simulink model "SCwith2SAs2aug"  (R2025b)
settings: Solver=VariableStepAuto  StartTime=0.0  StopTime=10.0  RelTol=1e-3
undefined symbols (not defined in the file or in its folder): DAP0, InvDyn, Jr, sig4, uls, ureal, uss, uw, XI
libraries: RCTblocks x77
(part 1 of 2)
settings Model: Creator=d.alazard  LastModifiedBy=andre
settings SolverCC: AlgebraicLoopSolver=TrustRegion
settings DebuggingCC: AlgebraicLoopMsg=none  UnconnectedInputMsg=warning  UnconnectedOutputMsg=warning  UnconnectedLineMsg=warning
settings ModelReferenceCC: EnableRefExpFcnMdlSchedulingChecks=on
settings RTWCC: GPUComputeCapability=3.5  DLArmComputeVersion=19.05

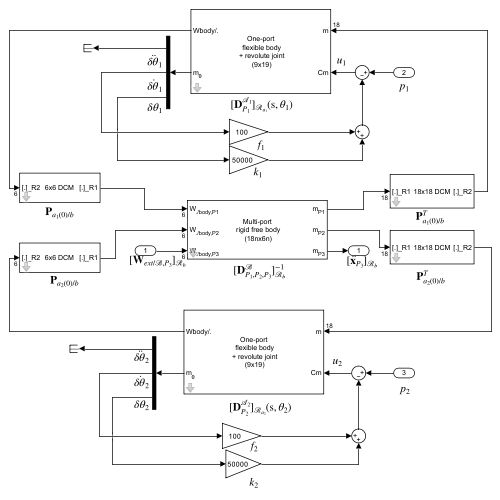
[thumbnail: Simulink's stored preview of the top-level diagram]
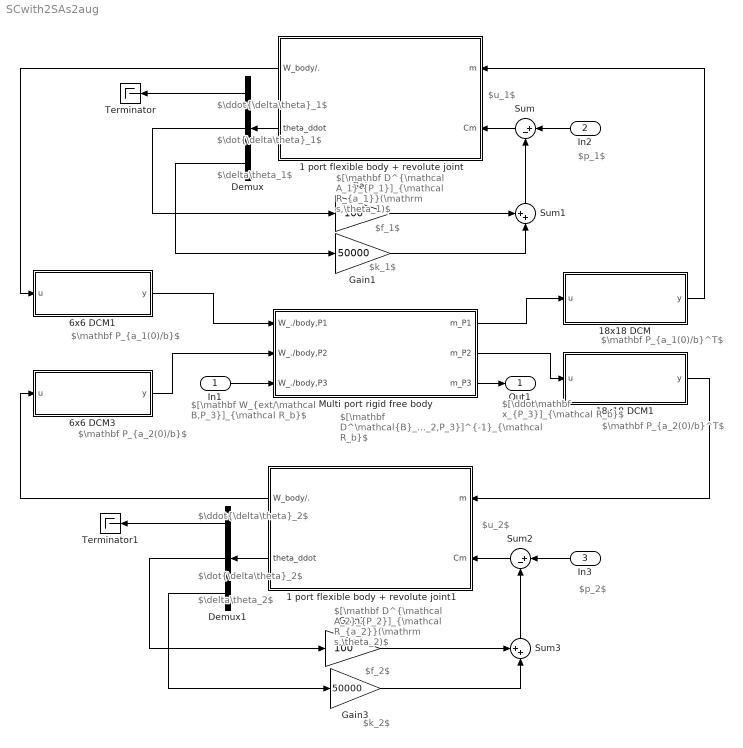
== system SCwith2SAs2aug ==
  note: $[\ddot\mathbf x_{P_3}]_{\mathcal R_b}$
  note: $u_1$
  note: $\ddot{\delta\theta}_1$
  note: $\mathbf P_{a_1(0)/b}^T$
  note: $[\mathbf D^\mathcal{B}_{P_1,P_2,P_3}]^{-1}_{\mathcal R_b}$
  note: $\mathbf P_{a_1(0)/b}$
  note: $\mathbf P_{a_2(0)/b}$
  note: $\mathbf P_{a_2(0)/b}^T$
  note: $\dot{\delta\theta}_1$
  note: $\dot{\delta\theta}_2$
  note: $\ddot{\delta\theta}_2$
  note: $\delta\theta_1$
  note: $\delta\theta_2$
  note: $p_1$
  note: $u_2$
  note: $p_2$
  note: $f_1$
  note: $k_1$
  note: $k_2$
  note: $f_2$
  note: $[\mathbf D^{\mathcal A_1}_{P_1}]_{\mathcal R_{a_1}}(\mathrm s,\theta_1)$
  note: $[\mathbf D^{\mathcal A_2}_{P_2}]_{\mathcal R_{a_2}}(\mathrm s,\theta_2)$
  note: $[\mathbf W_{ext/\mathcal B,P_3}]_{\mathcal R_b}$
  In1 : Inport
  In2 : Inport  Port=2
  In3 : Inport  Port=3
  1 port flexible body + revolute joint : Subsystem  mask(One-port flexibe body with revolute joint (9x19)){m=43, Ig=[17 0 0;0 62 0;0 0 79], OG=[2.07;0;0], OP=[0;0;0], ra=[1;0;0], theta=ureal('Theta',0,'Range',[-pi pi]), n=3, xi=0.005, w1=ureal('w1',5.6,'percent',20), L11=0, L12=0, L13=-5.12, L14=0, L15=12.5, L16=0, w2=ureal('w2',19.3,'percent',20), L21=0, L22=0, L23=0, L24=-3.84, L25=0, L26=0, w3=ureal('w3',35.4,'percent',20), L31=0, L32=0, L33=-2.97, L34=0, L35=2.51, L36=0, w4=2.83*2*pi, L41=0.0004, L42=-0.9132, L43=2.7900, L44=-1.8763, L45=-0.0246, L46=0.0031, w5=4.30*2*pi, L51=-0.0053, L52=5.878, L53=-1.0144, L54=3.0180, L55=-0.0124, L56=-0.0001, w6=0, L61=0, L62=0, L63=0, L64=0, L65=0, L66=0, w7=0, L71=0, L72=0, L73=0, L74=0, L75=0, L76=0, w8=0, L81=0, L82=0, L83=0, L84=0, L85=0, L86=0, w9=0, L91=0, L92=0, L93=0, L94=0, L95=0, L96=0, w10=0, L101=0, L102=0, L103=0, L104=0, L105=0, L106=0}
      mask prompts: m "Mass (Kg)"; Ig "Inertia (at G in Ra, Kgm^2)"; OG "OG (3x1 vector in Ra, m)"; OP "OP (3x1 vector in Ra, m)"; ra "ra (joint axis) (3x1 vector)"; theta "Angular configuration (rad)"; n "Number of flexible modes"; xi "Common damping ratio"; w1 "Frequency (rd/s)"; L11 "Tx (Kg^0.5)"; L12 "Ty (Kg^0.5)"; L13 "Tz (Kg^0.5)"; L14 "Rx (m.Kg^0.5)"; L15 "Ry (m.Kg^0.5)"; L16 "Rz (m.Kg^0.5)"; w2 "Frequency (rd/s)"; L21 "Tx (Kg^0.5)"; L22 "Ty (Kg^0.5)"; L23 "Tz (Kg^0.5)"; L24 "Rx (m.Kg^0.5)"; L25 "Ry (m.Kg^0.5)"; L26 "Rz (m.Kg^0.5)"; w3 "Frequency (rd/s)"; L31 "Tx (Kg^0.5)"; L32 "Ty (Kg^0.5)"; L33 "Tz (Kg^0.5)"; L34 "Rx (m.Kg^0.5)"; L35 "Ry (m.Kg^0.5)"; L36 "Rz (m.Kg^0.5)"; w4 "Frequency (rd/s)"; L41 "Tx (Kg^0.5)"; L42 "Ty (Kg^0.5)"; L43 "Tz (Kg^0.5)"; L44 "Rx (m.Kg^0.5)"; L45 "Ry (m.Kg^0.5)"; L46 "Rz (m.Kg^0.5)"; w5 "Frequency (rd/s)"; L51 "Tx (Kg^0.5)"; L52 "Ty (Kg^0.5)"; L53 "Tz (Kg^0.5)"; L54 "Rx (m.Kg^0.5)"; L55 "Ry (m.Kg^0.5)"; L56 "Rz (m.Kg^0.5)"; w6 "Frequency (rd/s)"; L61 "Tx (Kg^0.5)"; L62 "Ty (Kg^0.5)"; L63 "Tz (Kg^0.5)"; L64 "Rx (m.Kg^0.5)"; L65 "Ry (m.Kg^0.5)"; L66 "Rz (m.Kg^0.5)"; w7 "Frequency (rd/s)"; L71 "Tx (Kg^0.5)"; L72 "Ty (Kg^0.5)"; L73 "Tz (Kg^0.5)"; L74 "Rx (m.Kg^0.5)"; L75 "Ry (m.Kg^0.5)"; L76 "Rz (m.Kg^0.5)"; w8 "Frequency (rd/s)"; L81 "Tx (Kg^0.5)"; L82 "Ty (Kg^0.5)"; L83 "Tz (Kg^0.5)"; L84 "Rx (m.Kg^0.5)"; L85 "Ry (m.Kg^0.5)"; L86 "Rz (m.Kg^0.5)"; w9 "Frequency (rd/s)"; L91 "Tx (Kg^0.5)"; L92 "Ty (Kg^0.5)"; L93 "Tz (Kg^0.5)"; L94 "Rx (m.Kg^0.5)"; L95 "Ry (m.Kg^0.5)"; L96 "Rz (m.Kg^0.5)"; w10 "Frequency (rd/s)"; L101 "Tx (Kg^0.5)"; L102 "Ty (Kg^0.5)"; L103 "Tz (Kg^0.5)"; L104 "Rx (m.Kg^0.5)"; L105 "Ry (m.Kg^0.5)"; L106 "Rz (m.Kg^0.5)"
      mask help:
      | 9x19 dynamic model of a flexible body connected at point P to a parent body through a revolute joint:
      |  - 6x18 transfer from the motion vectort to the wrench applied by this body to the parent body at point P and
      |    projected in the parent body frame Rp.
      |  - the 3x1 channel  is the transfer:
      |               * from  the  joint torque applied by the input (parent) shaft to the output (body) shaft
      |               * to the relative motion vector of the output shaft w.r.t the input shaft [thetaddot;thetadot;theta].
      |
      | O: the body reference point
      | G: the center of mass
      | P: the connection point with a revolute joint
      | ra: direction of the revolute joint in the parent body frame Rp (or the flexible body frame Ra)
      |
      | All mechanical parameters are expressed in the flexible body frame Ra.
      | Each parameter can be an uncertain parameter declared with "ureal" (except ra)
      |
      | Angular configuration can be a vayring parameter: Ex:
      | ureal('NAME',0,'Range',[-pi pi])
      | Then, ULINEARIZE will provide a model involving the block named "tan_NAME_div4".
      mask init:
      | FlexBodyRev1Port
      mask Help: web('Doconeportflexrevolute.html','-browser')
      mask TypeOptions n: 0 | 1 | 2 | 3 | 4 | 5 | 6 | 7 | 8 | 9 | 10
      mask DialogControl ParameterGroupVar Prompt: Main parameters
      mask DialogControl damping Prompt: Damping ratio
      mask DialogControl mode1 Prompt: Flexible mode #1:
      mask DialogControl Control8 Prompt: Modal participation factor at P in Ra
      mask DialogControl mode2 Prompt: #2:
      mask DialogControl Control9 Prompt: Modal participation factor at P in Ra
      mask DialogControl mode3 Prompt: #3
      mask DialogControl Control10 Prompt: Modal participation factor at P in Ra
      mask DialogControl mode4 Prompt: #4
      mask DialogControl Control11 Prompt: Modal participation factor at P in Ra
      mask DialogControl mode5 Prompt: #5
      mask DialogControl Control12 Prompt: Modal participation factor at P in Ra
      mask DialogControl mode6 Prompt: #6
      mask DialogControl Control13 Prompt: Modal participation factor at P in Ra
      mask DialogControl mode7 Prompt: #7
      mask DialogControl Control14 Prompt: Modal participation factor at P in Ra
      mask DialogControl mode8 Prompt: #8
      mask DialogControl Control15 Prompt: Modal participation factor at P in Ra
      mask DialogControl mode9 Prompt: #9
      mask DialogControl Control16 Prompt: Modal participation factor at P in Ra
      mask DialogControl mode10 Prompt: #10
      mask DialogControl Control17 Prompt: Modal participation factor at P in Ra
      mask Display:
      | disp('One-port\n flexible body\n + revolute joint\n (9x19)')
      | port_label('input', 1, 'm')
      | port_label('output', 1, 'Wbody/.')
      | port_label('input', 2, 'Cm')
      | port_label('output', 2, 'm_\theta','interpreter','tex')
  1 port flexible body + revolute joint1 : Subsystem  mask(One-port flexibe body with revolute joint (9x19)){m=43, Ig=[17 0 0;0 62 0;0 0 79], OG=[2.07;0;0], OP=[0;0;0], ra=[-1;0;0], theta=ureal('Theta',0,'Range',[-pi pi]), n=3, xi=0.005, w1=ureal('w1',5.6,'percent',20), L11=0, L12=0, L13=-5.12, L14=0, L15=12.5, L16=0, w2=ureal('w2',19.3,'percent',20), L21=0, L22=0, L23=0, L24=-3.84, L25=0, L26=0, w3=ureal('w3',35.4,'percent',20), L31=0, L32=0, L33=-2.97, L34=0, L35=2.51, L36=0, w4=2.83*2*pi, L41=0.0004, L42=-0.9132, L43=2.7900, L44=-1.8763, L45=-0.0246, L46=0.0031, w5=4.30*2*pi, L51=-0.0053, L52=5.878, L53=-1.0144, L54=3.0180, L55=-0.0124, L56=-0.0001, w6=0, L61=0, L62=0, L63=0, L64=0, L65=0, L66=0, w7=0, L71=0, L72=0, L73=0, L74=0, L75=0, L76=0, w8=0, L81=0, L82=0, L83=0, L84=0, L85=0, L86=0, w9=0, L91=0, L92=0, L93=0, L94=0, L95=0, L96=0, w10=0, L101=0, L102=0, L103=0, L104=0, L105=0, L106=0}
      mask prompts: m "Mass (Kg)"; Ig "Inertia (at G in Ra, Kgm^2)"; OG "OG (3x1 vector in Ra, m)"; OP "OP (3x1 vector in Ra, m)"; ra "ra (joint axis) (3x1 vector)"; theta "Angular configuration (rad)"; n "Number of flexible modes"; xi "Common damping ratio"; w1 "Frequency (rd/s)"; L11 "Tx (Kg^0.5)"; L12 "Ty (Kg^0.5)"; L13 "Tz (Kg^0.5)"; L14 "Rx (m.Kg^0.5)"; L15 "Ry (m.Kg^0.5)"; L16 "Rz (m.Kg^0.5)"; w2 "Frequency (rd/s)"; L21 "Tx (Kg^0.5)"; L22 "Ty (Kg^0.5)"; L23 "Tz (Kg^0.5)"; L24 "Rx (m.Kg^0.5)"; L25 "Ry (m.Kg^0.5)"; L26 "Rz (m.Kg^0.5)"; w3 "Frequency (rd/s)"; L31 "Tx (Kg^0.5)"; L32 "Ty (Kg^0.5)"; L33 "Tz (Kg^0.5)"; L34 "Rx (m.Kg^0.5)"; L35 "Ry (m.Kg^0.5)"; L36 "Rz (m.Kg^0.5)"; w4 "Frequency (rd/s)"; L41 "Tx (Kg^0.5)"; L42 "Ty (Kg^0.5)"; L43 "Tz (Kg^0.5)"; L44 "Rx (m.Kg^0.5)"; L45 "Ry (m.Kg^0.5)"; L46 "Rz (m.Kg^0.5)"; w5 "Frequency (rd/s)"; L51 "Tx (Kg^0.5)"; L52 "Ty (Kg^0.5)"; L53 "Tz (Kg^0.5)"; L54 "Rx (m.Kg^0.5)"; L55 "Ry (m.Kg^0.5)"; L56 "Rz (m.Kg^0.5)"; w6 "Frequency (rd/s)"; L61 "Tx (Kg^0.5)"; L62 "Ty (Kg^0.5)"; L63 "Tz (Kg^0.5)"; L64 "Rx (m.Kg^0.5)"; L65 "Ry (m.Kg^0.5)"; L66 "Rz (m.Kg^0.5)"; w7 "Frequency (rd/s)"; L71 "Tx (Kg^0.5)"; L72 "Ty (Kg^0.5)"; L73 "Tz (Kg^0.5)"; L74 "Rx (m.Kg^0.5)"; L75 "Ry (m.Kg^0.5)"; L76 "Rz (m.Kg^0.5)"; w8 "Frequency (rd/s)"; L81 "Tx (Kg^0.5)"; L82 "Ty (Kg^0.5)"; L83 "Tz (Kg^0.5)"; L84 "Rx (m.Kg^0.5)"; L85 "Ry (m.Kg^0.5)"; L86 "Rz (m.Kg^0.5)"; w9 "Frequency (rd/s)"; L91 "Tx (Kg^0.5)"; L92 "Ty (Kg^0.5)"; L93 "Tz (Kg^0.5)"; L94 "Rx (m.Kg^0.5)"; L95 "Ry (m.Kg^0.5)"; L96 "Rz (m.Kg^0.5)"; w10 "Frequency (rd/s)"; L101 "Tx (Kg^0.5)"; L102 "Ty (Kg^0.5)"; L103 "Tz (Kg^0.5)"; L104 "Rx (m.Kg^0.5)"; L105 "Ry (m.Kg^0.5)"; L106 "Rz (m.Kg^0.5)"
      mask help:
      | 9x19 dynamic model of a flexible body connected at point P to a parent body through a revolute joint:
      |  - 6x18 transfer from the motion vectort to the wrench applied by this body to the parent body at point P and
      |    projected in the parent body frame Rp.
      |  - the 3x1 channel  is the transfer:
      |               * from  the  joint torque applied by the input (parent) shaft to the output (body) shaft
      |               * to the relative motion vector of the output shaft w.r.t the input shaft [thetaddot;thetadot;theta].
      |
      | O: the body reference point
      | G: the center of mass
      | P: the connection point with a revolute joint
      | ra: direction of the revolute joint in the parent body frame Rp (or the flexible body frame Ra)
      |
      | All mechanical parameters are expressed in the flexible body frame Ra.
      | Each parameter can be an uncertain parameter declared with "ureal" (except ra)
      |
      | Angular configuration can be a vayring parameter: Ex:
      | ureal('NAME',0,'Range',[-pi pi])
      | Then, ULINEARIZE will provide a model involving the block named "tan_NAME_div4".
      mask init:
      | FlexBodyRev1Port
      mask Help: web('Doconeportflexrevolute.html','-browser')
      mask TypeOptions n: 0 | 1 | 2 | 3 | 4 | 5 | 6 | 7 | 8 | 9 | 10
      mask DialogControl ParameterGroupVar Prompt: Main parameters
      mask DialogControl damping Prompt: Damping ratio
      mask DialogControl mode1 Prompt: Flexible mode #1:
      mask DialogControl Control8 Prompt: Modal participation factor at P in Ra
      mask DialogControl mode2 Prompt: #2:
      mask DialogControl Control9 Prompt: Modal participation factor at P in Ra
      mask DialogControl mode3 Prompt: #3
      mask DialogControl Control10 Prompt: Modal participation factor at P in Ra
      mask DialogControl mode4 Prompt: #4
      mask DialogControl Control11 Prompt: Modal participation factor at P in Ra
      mask DialogControl mode5 Prompt: #5
      mask DialogControl Control12 Prompt: Modal participation factor at P in Ra
      mask DialogControl mode6 Prompt: #6
      mask DialogControl Control13 Prompt: Modal participation factor at P in Ra
      mask DialogControl mode7 Prompt: #7
      mask DialogControl Control14 Prompt: Modal participation factor at P in Ra
      mask DialogControl mode8 Prompt: #8
      mask DialogControl Control15 Prompt: Modal participation factor at P in Ra
      mask DialogControl mode9 Prompt: #9
      mask DialogControl Control16 Prompt: Modal participation factor at P in Ra
      mask DialogControl mode10 Prompt: #10
      mask DialogControl Control17 Prompt: Modal participation factor at P in Ra
      mask Display:
      | disp('One-port\n flexible body\n + revolute joint\n (9x19)')
      | port_label('input', 1, 'm')
      | port_label('output', 1, 'Wbody/.')
      | port_label('input', 2, 'Cm')
      | port_label('output', 2, 'm_\theta','interpreter','tex')
  18x18 DCM : Subsystem  mask(18x18 Direction cosine matrix (DCM)){rot=[0 -1 0;0 0 -1;1 0 0], transp=on}
      mask prompts: rot "3x3 DCM"; transp "Matrix transposed"
      mask help:
      | For 6 d.o.f. body motion vector (3 translations and 3 rotations, accelerations, velocities and positions), this block Implement the 18x18 rotation matrix (or its transposed) for a given 3x3 DCM.
      |
      | Considering 2 frames R1 and  R2, the DCM between R1 and R2 is defined as the 3x3 matrix where each column is the component vector of each R2 orthogonal unit vector expressed in R1. Thus
      |
      |    [v]_R1 = DCM  * [v]_R2.
      mask init:
      | if transp,
      |     rot=rot';
      | end
      mask Help: web('Doc18dcm.html','-browser')
      mask Display:
      | disp('18x18 DCM')
      | if transp
      |     port_label('input', 1, '[.]_R1')
      |     port_label('output', 1, '[.]_R2')
      | else
      |     port_label('input', 1, '[.]_R2')
      |     port_label('output', 1, '[.]_R1')
      | end
  18x18 DCM1 : Subsystem  mask(18x18 Direction cosine matrix (DCM)){rot=[0 1 0;0 0 -1;-1 0 0], transp=on}
      mask prompts: rot "3x3 DCM"; transp "Matrix transposed"
      mask help:
      | For 6 d.o.f. body motion vector (3 translations and 3 rotations, accelerations, velocities and positions), this block Implement the 18x18 rotation matrix (or its transposed) for a given 3x3 DCM.
      |
      | Considering 2 frames R1 and  R2, the DCM between R1 and R2 is defined as the 3x3 matrix where each column is the component vector of each R2 orthogonal unit vector expressed in R1. Thus
      |
      |    [v]_R1 = DCM  * [v]_R2.
      mask init:
      | if transp,
      |     rot=rot';
      | end
      mask Help: web('Doc18dcm.html','-browser')
      mask Display:
      | disp('18x18 DCM')
      | if transp
      |     port_label('input', 1, '[.]_R1')
      |     port_label('output', 1, '[.]_R2')
      | else
      |     port_label('input', 1, '[.]_R2')
      |     port_label('output', 1, '[.]_R1')
      | end
  6x6 DCM1 : Subsystem  mask(6x6 Direction cosine matrix (DCM)){rot=[0 -1 0;0 0 -1;1 0 0], transp=off}
      mask prompts: rot "3x3 DCM"; transp "Matrix transposed"
      mask help:
      | For 6 d.o.f. body motion (3 translations and 3 rotations), this block Implement the 6x6 rotation matrix (or its transposed) for a given 3x3 DCM.
      |
      | Considering 2 frames R1 and  R2, the DCM between R1 and R2 is defined as the 3x3 matrix where each column is the component vector of each R2 orthogonal unit vector expressed in R1. Thus
      |
      |    [v]_R1 = DCM  * [v]_R2.
      mask init:
      | if transp,
      |     rot=rot';
      | end
      mask Help: web('Doc6dcm.html','-browser')
      mask Display:
      | disp('6x6 DCM')
      | if transp
      |     port_label('input', 1, '[.]_R1')
      |     port_label('output', 1, '[.]_R2')
      | else
      |     port_label('input', 1, '[.]_R2')
      |     port_label('output', 1, '[.]_R1')
      | end
  6x6 DCM3 : Subsystem  mask(6x6 Direction cosine matrix (DCM)){rot=[0 1 0;0 0 -1;-1 0 0], transp=off}
      mask prompts: rot "3x3 DCM"; transp "Matrix transposed"
      mask help:
      | For 6 d.o.f. body motion (3 translations and 3 rotations), this block Implement the 6x6 rotation matrix (or its transposed) for a given 3x3 DCM.
      |
      | Considering 2 frames R1 and  R2, the DCM between R1 and R2 is defined as the 3x3 matrix where each column is the component vector of each R2 orthogonal unit vector expressed in R1. Thus
      |
      |    [v]_R1 = DCM  * [v]_R2.
      mask init:
      | if transp,
      |     rot=rot';
      | end
      mask Help: web('Doc6dcm.html','-browser')
      mask Display:
      | disp('6x6 DCM')
      | if transp
      |     port_label('input', 1, '[.]_R1')
      |     port_label('output', 1, '[.]_R2')
      | else
      |     port_label('input', 1, '[.]_R2')
      |     port_label('output', 1, '[.]_R1')
      | end
  Demux : Demux  Outputs=3
  Demux1 : Demux  Outputs=3
  Gain : Gain  Gain=100
  Gain1 : Gain  Gain=50000
  Gain2 : Gain  Gain=100
  Gain3 : Gain  Gain=50000
  Multi port rigid free body : Subsystem  mask(Multi-port rigid body (18nx6n)){m=ureal('mB',1000,'percent',20), Ig=[ureal('IBx',75,'percent',20) 1 2;1 ureal('IBy',40,'percent',20) -1;2 -1 ureal('IBz',80,'percent',20)], OG=[0.35;1.5;0.5], n=3, OP1=[0.4;1.4;1], OP2=[0.4;1.4;0], OP3=[0.35;1.5;0.5], OP4=[0;0;0], OP5=[0;0;0]}
      mask prompts: m "Mass (Kg)"; Ig "Inertia (at G, Kg m^2)"; OG "OG (3x1 vector, m)"; n "Number of ports"; OP1 "OP1 (3x1 vector, m)"; OP2 "OP2 (3x1 vector, m)"; OP3 "OP3 (3x1 vector, m)"; OP4 "OP4 (3x1 vector, m)"; OP5 "OP5 (3x1 vector,m)"
      mask help:
      | 18nx6n dynamic model of a rigid body at n given points (ports) between wrenches applied at the n points (input) and the motions vectors at these points (output).
      |
      | 0: the reference point
      | G: the center of mass
      | Pi (i=1:n): the n given connection points (n<6).
      |
      | All parameters are expressed in the body frame.
      | Each parameter can be an uncertain parameter declared with "ureal"
      mask init:
      | MultiPortRigidFreeBody
      mask Help: web('Docmultiportrigidbase.html','-browser')
      mask TypeOptions n: 1 | 2 | 3 | 4 | 5
      mask DialogControl ParameterGroupVar Prompt: Main parameters
      mask DialogControl port1 Prompt: Port #1
      mask DialogControl port2 Prompt: #2
      mask DialogControl port3 Prompt: #3
      mask DialogControl port4 Prompt: #4
      mask DialogControl port5 Prompt: #5
      mask Display:
      | disp('Multi-port\n rigid free body\n (18nx6n)')
      | for ii=1:n
      |     port_label('input', ii,['W_{./body,P',num2str(ii),'}'],'interpreter','tex')
      |     port_label('output',ii,['m_{P',num2str(ii),'}'],'interpreter','tex')
      | end
  Sum : Sum  Inputs=|+-
  Sum1 : Sum  Inputs=++|
  Sum2 : Sum  Inputs=|+-
  Sum3 : Sum  Inputs=++|
  Terminator : Terminator
  Terminator1 : Terminator
  Out1 : Outport
  wires:
  6x6 DCM1/1(y) -> Multi port rigid free body/1(W_./body,P1)
  Multi port rigid free body/1(m_P1) -> 18x18 DCM/1(u)
  6x6 DCM3/1(y) -> Multi port rigid free body/2(W_./body,P2)
  Multi port rigid free body/2(m_P2) -> 18x18 DCM1/1(u)
  18x18 DCM/1(y) -> 1 port flexible body + revolute joint/1(m)
  1 port flexible body + revolute joint/1(W_body/.) -> 6x6 DCM1/1(u)
  18x18 DCM1/1(y) -> 1 port flexible body + revolute joint1/1(m)
  1 port flexible body + revolute joint1/1(W_body/.) -> 6x6 DCM3/1(u)
  In1/1 -> Multi port rigid free body/3(W_./body,P3)
  Multi port rigid free body/3(m_P3) -> Out1/1
  Demux/3 -> Gain1/1
  In2/1 -> Sum/1
  Gain/1 -> Sum1/1
  Gain1/1 -> Sum1/2
  Sum1/1 -> Sum/2
  Sum/1 -> 1 port flexible body + revolute joint/2(Cm)
  Gain2/1 -> Sum3/1
  Sum3/1 -> Sum2/2
  In3/1 -> Sum2/1
  Sum2/1 -> 1 port flexible body + revolute joint1/2(Cm)
  Gain3/1 -> Sum3/2
  1 port flexible body + revolute joint/2(theta_ddot) -> Demux/1
  Demux/2 -> Gain/1
  Demux/1 -> Terminator/1
  Demux1/1 -> Terminator1/1
  1 port flexible body + revolute joint1/2(theta_ddot) -> Demux1/1
  Demux1/3 -> Gain3/1
  Demux1/2 -> Gain2/1

== system SCwith2SAs2aug/1 port flexible body + revolute joint ==
  m : Inport  PortDimensions=18
  Cm : Inport  Port=2  PortDimensions=1
  2*xi diagonal matrix : RCTblocks/Uncertain State Space  Tag=USS  USystem=uss(2*XI)  UValue=[]  X0=[]  uX0=[]
  Add : Sum  Inputs=--
  Add1 : Sum
  Add2 : Sum  Inputs=+-
  DAP0 : RCTblocks/Uncertain State Space  Tag=USS  USystem=uss(DAP0)  UValue=[]  X0=[]  uX0=[]
  Demux : Demux  Outputs=[6 12]
  Integrator : Integrator
  Integrator1 : Integrator
  Revolute joint + configuration : Subsystem  mask(Revolute joint){ra=ra, Jr=Jr, theta=theta}
      mask prompts: ra "Direction of the joint in the local frame (3x1 vector)"; Jr "Rotor inertia (kg.m^2)"; theta "Angular configuration (rad)"
      mask help:
      | This block implement the TITOP model of of a revolute joint.
      | The last channel is the transfer between the torque applied inside the joint by the input shaft to the output shaft and the relative angular acceleration of the output shaft w.r.t the input shaft.
      |
      | Angular configuration can be a vayring parameter: Ex:
      | ureal('NAME',0,'Range',[-pi pi])
      |
      | Then, ULINEARIZE will provide a model involving the block named "tan_NAME_div4";
      mask init:
      | pass=ra2DCMi(ra);
      | ran=[ra(1);ra(2);ra(3)]/norm(ra);
      mask Help: web('DocRevoluteJoint_configuration.html','-browser')
      mask Display:
      | disp('Revolute joint\nTITOP model\n+ angle configuration')
      | port_label('input', 1, 'W_./r_out|a')
      | port_label('output', 1, 'm_out|a')
      | port_label('input', 2, 'm_in|p')
      | port_label('output', 2, 'W_r_in/.|p')
      | port_label('input', 3, 'Cm')
      | port_label('output', 3, 'm_\theta','interpreter','tex')
  Terminator : Terminator
  "[Lp] ' Ra" : RCTblocks/Uncertain State Space  Tag=USS  USystem=uss(uls')  UValue=[]  X0=[]  uX0=[]
  "[Lp] Ra" : RCTblocks/Uncertain State Space  Tag=USS  USystem=uss(uls)  UValue=[]  X0=[]  uX0=[]
  omega diagonal matrix : RCTblocks/Uncertain State Space  Tag=USS  USystem=uss(diag(uw))  UValue=[]  X0=[]  uX0=[]
  omega diagonal matrix. : RCTblocks/Uncertain State Space  Tag=USS  USystem=uss(diag(uw))  UValue=[]  X0=[]  uX0=[]
  W_body/. : Outport  VectorParamsAs1DForOutWhenUnconnected=off
  theta_ddot : Outport  Port=2  VectorParamsAs1DForOutWhenUnconnected=off
  wires:
  Demux/2 -> Terminator/1
  Demux/1 -> DAP0/1, "[Lp] Ra"/1  "[ Xddot(p) ]/Ra"
  Revolute joint + configuration/1(m_out|a) -> Demux/1
  Revolute joint + configuration/3(m_theta) -> theta_ddot/1
  Cm/1 -> Revolute joint + configuration/3(Cm)
  Revolute joint + configuration/2(W_r_in/.|p) -> W_body/./1
  m/1 -> Revolute joint + configuration/2(m_in|p)
  DAP0/1 -> Add2/2
  "[Lp] ' Ra"/1 -> Add2/1
  omega diagonal matrix./1 -> Add1/1
  Integrator/1 -> 2*xi diagonal matrix/1, Integrator1/1  "eta dot"
  Integrator1/1 -> omega diagonal matrix./1  "eta"
  Add/1 -> Integrator/1  "eta dot dot"
  Add1/1 -> omega diagonal matrix/1
  2*xi diagonal matrix/1 -> Add1/2
  "[Lp] Ra"/1 -> Add/2
  omega diagonal matrix/1 -> "[Lp] ' Ra"/1, Add/1
  Add2/1 -> Revolute joint + configuration/1(W_./r_out|a)  "[ F(A/P,p) ]/Ra"

== system SCwith2SAs2aug/1 port flexible body + revolute joint1 ==
  m : Inport  PortDimensions=18
  Cm : Inport  Port=2  PortDimensions=1
  2*xi diagonal matrix : RCTblocks/Uncertain State Space  Tag=USS  USystem=uss(2*XI)  UValue=[]  X0=[]  uX0=[]
  Add : Sum  Inputs=--
  Add1 : Sum
  Add2 : Sum  Inputs=+-
  DAP0 : RCTblocks/Uncertain State Space  Tag=USS  USystem=uss(DAP0)  UValue=[]  X0=[]  uX0=[]
  Demux : Demux  Outputs=[6 12]
  Integrator : Integrator
  Integrator1 : Integrator
  Revolute joint + configuration : Subsystem  mask(Revolute joint){ra=ra, Jr=Jr, theta=theta}
      mask prompts: ra "Direction of the joint in the local frame (3x1 vector)"; Jr "Rotor inertia (kg.m^2)"; theta "Angular configuration (rad)"
      mask help:
      | This block implement the TITOP model of of a revolute joint.
      | The last channel is the transfer between the torque applied inside the joint by the input shaft to the output shaft and the relative angular acceleration of the output shaft w.r.t the input shaft.
      |
      | Angular configuration can be a vayring parameter: Ex:
      | ureal('NAME',0,'Range',[-pi pi])
      |
      | Then, ULINEARIZE will provide a model involving the block named "tan_NAME_div4";
      mask init:
      | pass=ra2DCMi(ra);
      | ran=[ra(1);ra(2);ra(3)]/norm(ra);
      mask Help: web('DocRevoluteJoint_configuration.html','-browser')
      mask Display:
      | disp('Revolute joint\nTITOP model\n+ angle configuration')
      | port_label('input', 1, 'W_./r_out|a')
      | port_label('output', 1, 'm_out|a')
      | port_label('input', 2, 'm_in|p')
      | port_label('output', 2, 'W_r_in/.|p')
      | port_label('input', 3, 'Cm')
      | port_label('output', 3, 'm_\theta','interpreter','tex')
  Terminator : Terminator
  "[Lp] ' Ra" : RCTblocks/Uncertain State Space  Tag=USS  USystem=uss(uls')  UValue=[]  X0=[]  uX0=[]
  "[Lp] Ra" : RCTblocks/Uncertain State Space  Tag=USS  USystem=uss(uls)  UValue=[]  X0=[]  uX0=[]
  omega diagonal matrix : RCTblocks/Uncertain State Space  Tag=USS  USystem=uss(diag(uw))  UValue=[]  X0=[]  uX0=[]
  omega diagonal matrix. : RCTblocks/Uncertain State Space  Tag=USS  USystem=uss(diag(uw))  UValue=[]  X0=[]  uX0=[]
  W_body/. : Outport  VectorParamsAs1DForOutWhenUnconnected=off
  theta_ddot : Outport  Port=2  VectorParamsAs1DForOutWhenUnconnected=off
  wires:
  Add2/1 -> Revolute joint + configuration/1(W_./r_out|a)  "[ F(A/P,p) ]/Ra"
  omega diagonal matrix/1 -> Add/1, "[Lp] ' Ra"/1
  "[Lp] Ra"/1 -> Add/2
  2*xi diagonal matrix/1 -> Add1/2
  Add1/1 -> omega diagonal matrix/1
  Add/1 -> Integrator/1  "eta dot dot"
  Integrator1/1 -> omega diagonal matrix./1  "eta"
  Integrator/1 -> Integrator1/1, 2*xi diagonal matrix/1  "eta dot"
  omega diagonal matrix./1 -> Add1/1
  "[Lp] ' Ra"/1 -> Add2/1
  DAP0/1 -> Add2/2
  m/1 -> Revolute joint + configuration/2(m_in|p)
  Revolute joint + configuration/2(W_r_in/.|p) -> W_body/./1
  Cm/1 -> Revolute joint + configuration/3(Cm)
  Revolute joint + configuration/3(m_theta) -> theta_ddot/1
  Revolute joint + configuration/1(m_out|a) -> Demux/1
  Demux/1 -> "[Lp] Ra"/1, DAP0/1  "[ Xddot(p) ]/Ra"
  Demux/2 -> Terminator/1

== system SCwith2SAs2aug/18x18 DCM ==
  u : Inport  PortDimensions=18
  Demux : Demux  Outputs=[3 3 3 3 3 3]
  Mux : Mux  Inputs=[3 3 3 3 3 3]
  rotation : Gain  Gain=rot  Multiplication=Matrix(K*u) (u vector)
  rotation1 : Gain  Gain=rot  Multiplication=Matrix(K*u) (u vector)
  rotation2 : Gain  Gain=rot  Multiplication=Matrix(K*u) (u vector)
  translation : Gain  Gain=rot  Multiplication=Matrix(K*u) (u vector)
  translation1 : Gain  Gain=rot  Multiplication=Matrix(K*u) (u vector)
  translation2 : Gain  Gain=rot  Multiplication=Matrix(K*u) (u vector)
  y : Outport  VectorParamsAs1DForOutWhenUnconnected=off
  wires:
  Demux/6 -> rotation2/1
  rotation2/1 -> Mux/6
  translation2/1 -> Mux/5
  Demux/5 -> translation2/1
  rotation1/1 -> Mux/4
  translation1/1 -> Mux/3
  Demux/3 -> translation1/1
  Demux/4 -> rotation1/1
  Demux/2 -> rotation/1
  Mux/1 -> y/1
  u/1 -> Demux/1
  Demux/1 -> translation/1
  translation/1 -> Mux/1
  rotation/1 -> Mux/2

== system SCwith2SAs2aug/18x18 DCM1 ==
  u : Inport  PortDimensions=18
  Demux : Demux  Outputs=[3 3 3 3 3 3]
  Mux : Mux  Inputs=[3 3 3 3 3 3]
  rotation : Gain  Gain=rot  Multiplication=Matrix(K*u) (u vector)
  rotation1 : Gain  Gain=rot  Multiplication=Matrix(K*u) (u vector)
  rotation2 : Gain  Gain=rot  Multiplication=Matrix(K*u) (u vector)
  translation : Gain  Gain=rot  Multiplication=Matrix(K*u) (u vector)
  translation1 : Gain  Gain=rot  Multiplication=Matrix(K*u) (u vector)
  translation2 : Gain  Gain=rot  Multiplication=Matrix(K*u) (u vector)
  y : Outport  VectorParamsAs1DForOutWhenUnconnected=off
  wires:
  Demux/6 -> rotation2/1
  rotation2/1 -> Mux/6
  translation2/1 -> Mux/5
  Demux/5 -> translation2/1
  rotation1/1 -> Mux/4
  translation1/1 -> Mux/3
  Demux/3 -> translation1/1
  Demux/4 -> rotation1/1
  Demux/2 -> rotation/1
  Mux/1 -> y/1
  u/1 -> Demux/1
  Demux/1 -> translation/1
  translation/1 -> Mux/1
  rotation/1 -> Mux/2

== system SCwith2SAs2aug/6x6 DCM1 ==
  u : Inport  PortDimensions=6
  Demux : Demux  Outputs=[3 3]
  Mux : Mux  Inputs=[3 3]
  rotation : Gain  Gain=rot  Multiplication=Matrix(K*u) (u vector)
  translation : Gain  Gain=rot  Multiplication=Matrix(K*u) (u vector)
  y : Outport  VectorParamsAs1DForOutWhenUnconnected=off
  wires:
  rotation/1 -> Mux/2
  translation/1 -> Mux/1
  Demux/1 -> translation/1
  u/1 -> Demux/1
  Mux/1 -> y/1
  Demux/2 -> rotation/1

== system SCwith2SAs2aug/6x6 DCM3 ==
  u : Inport  PortDimensions=6
  Demux : Demux  Outputs=[3 3]
  Mux : Mux  Inputs=[3 3]
  rotation : Gain  Gain=rot  Multiplication=Matrix(K*u) (u vector)
  translation : Gain  Gain=rot  Multiplication=Matrix(K*u) (u vector)
  y : Outport  VectorParamsAs1DForOutWhenUnconnected=off
  wires:
  rotation/1 -> Mux/2
  translation/1 -> Mux/1
  Demux/1 -> translation/1
  u/1 -> Demux/1
  Mux/1 -> y/1
  Demux/2 -> rotation/1

== system SCwith2SAs2aug/Multi port rigid free body ==
  W_./body,P1 : Inport  PortDimensions=6
  W_./body,P2 : Inport  Port=2  PortDimensions=6
  W_./body,P3 : Inport  Port=3  PortDimensions=6
  Demux : Demux  Outputs=[18 18 18]
      settings: DisplayOption=none
  Gain : RCTblocks/Uncertain State Space  Tag=USS  USystem=uss(InvDyn)  UValue=[]  X0=[]  uX0=[]
  Mux : Mux  Inputs=[6 6 6]
  m_P1 : Outport
  m_P2 : Outport  Port=2
  m_P3 : Outport  Port=3
  wires:
  Demux/3 -> m_P3/1
  W_./body,P3/1 -> Mux/3
  Demux/2 -> m_P2/1
  W_./body,P2/1 -> Mux/2
  Demux/1 -> m_P1/1
  W_./body,P1/1 -> Mux/1
  Gain/1 -> Demux/1
  Mux/1 -> Gain/1

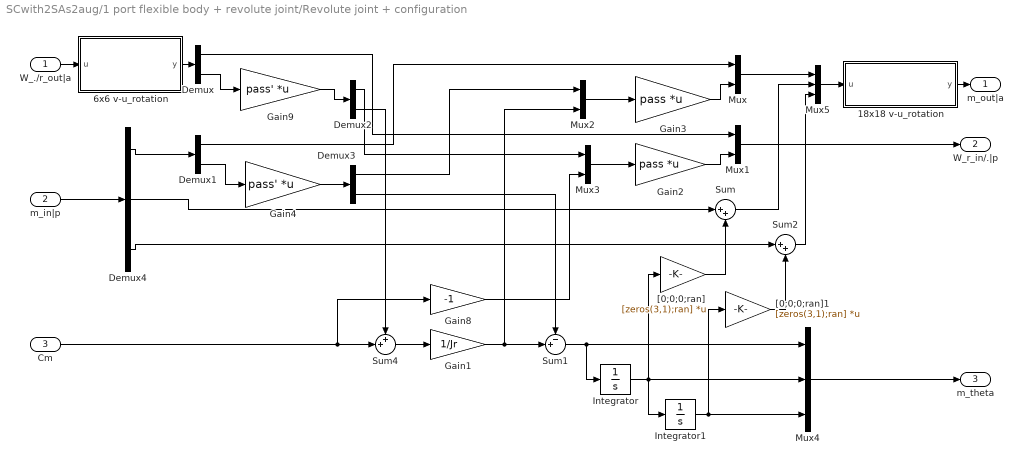
== system SCwith2SAs2aug/1 port flexible body + revolute joint/Revolute joint + configuration ==
  W_./r_out|a : Inport  PortDimensions=6
  m_in|p : Inport  Port=2  PortDimensions=18
  Cm : Inport  Port=3  PortDimensions=1
  18x18 v-u_rotation : Subsystem  mask(18x18 rotation matrix (around a given axis)){ra=ra, theta=theta, transp=on}
      mask prompts: ra "Rotation axis (3x1 vector)"; theta "Angle (rad)"; transp "Matrix transposed"
      mask help:
      | For 6 d.o.f. body motion vector (3 translations and 3 rotations, acceleration velocities and positions), this block Implement the 18x18 rotation matrix (or its transposed)  for a given angle around a given axis.
      |
      | Angle  (rad) can be an uncertain parameter declared with "ureal" with mode 'Range'
      | Ex: ureal('NAME',0,'Range',[-pi pi])
      | Then, ULINEARIZE will provide a model involving the block named "tan_NAME_div4".
      mask init:
      | vUrotation3x3
      mask Help: web('Doc6vurotation.html','-browser')
      mask Display:
      | disp('v-rot\n18x18')
      | if transp
      |     port_label('input', 1, '[.]_R1')
      |     port_label('output', 1, '[.]_R2')
      | else
      |     port_label('input', 1, '[.]_R2')
      |     port_label('output', 1, '[.]_R1')
      | end
  6x6 v-u_rotation : Subsystem  mask(6x6 rotation matrix (around a given axis)){ra=ra, theta=theta, transp=off}
      mask prompts: ra "Rotation axis (3x1 vector)"; theta "Angle (rad)"; transp "Matrix transposed"
      mask help:
      | For 6 d.o.f. body motion (3 translations and 3 rotations), this block Implement the 6x6 rotation matrix (or its transposed) for a given angle around a given axis.
      |
      | Angle  (rad) can be an uncertain parameter declared with "ureal" with mode 'Range'
      | Ex: ureal('NAME',0,'Range',[-pi pi])
      | Then, ULINEARIZE will provide a model involving the block named "tan_NAME_div4".
      mask init:
      | vUrotation3x3
      mask Help: web('Doc6vurotation.html','-browser')
      mask Display:
      | disp('v-rot\n6x6')
      | if transp
      |     port_label('input', 1, '[.]_R1')
      |     port_label('output', 1, '[.]_R2')
      | else
      |     port_label('input', 1, '[.]_R2')
      |     port_label('output', 1, '[.]_R1')
      | end
  Demux : Demux  Outputs=[3 3]
  Demux1 : Demux  Outputs=[3 3]
  Demux2 : Demux  Outputs=[2 1]
  Demux3 : Demux  Outputs=[2 1]
  Demux4 : Demux  Outputs=[6 6 6]
  Gain1 : Gain  Gain=1/Jr
  Gain2 : Gain  Gain=pass  Multiplication=Matrix(K*u) (u vector)
  Gain3 : Gain  Gain=pass  Multiplication=Matrix(K*u) (u vector)
  Gain4 : Gain  Gain=pass'  Multiplication=Matrix(K*u) (u vector)
  Gain8 : Gain  Gain=-1
  Gain9 : Gain  Gain=pass'  Multiplication=Matrix(K*u) (u vector)
  Integrator : Integrator
  Integrator1 : Integrator
  Mux : Mux  Inputs=[3 3]
  Mux1 : Mux  Inputs=[3 3]
  Mux2 : Mux  Inputs=[2 1]
  Mux3 : Mux  Inputs=[2 1]
  Mux4 : Mux  Inputs=3
  Mux5 : Mux  Inputs=[6 6 6]
  Sum : Sum  Inputs=|++
  Sum1 : Sum  Inputs=-+|
  Sum2 : Sum  Inputs=|++
  Sum4 : Sum  Inputs=++|
  "[0;0;0;ran]" : Gain  Gain=[zeros(3,1);ran]  Multiplication=Matrix(K*u) (u vector)
  "[0;0;0;ran]1" : Gain  Gain=[zeros(3,1);ran]  Multiplication=Matrix(K*u) (u vector)
  m_out|a : Outport  VectorParamsAs1DForOutWhenUnconnected=off
  W_r_in/.|p : Outport  Port=2  VectorParamsAs1DForOutWhenUnconnected=off
  m_theta : Outport  Port=3  VectorParamsAs1DForOutWhenUnconnected=off
  wires:
  Sum2/1 -> Mux5/3
  Sum/1 -> Mux5/2
  Mux5/1 -> 18x18 v-u_rotation/1(u)
  Mux/1 -> Mux5/1
  Demux4/3 -> Sum2/1
  Demux4/2 -> Sum/1
  "[0;0;0;ran]1"/1 -> Sum2/2
  "[0;0;0;ran]"/1 -> Sum/2
  Integrator1/1 -> Mux4/3, "[0;0;0;ran]1"/1
  Sum1/1 -> Mux4/1, Integrator/1
  Mux4/1 -> m_theta/1
  Integrator/1 -> Integrator1/1, Mux4/2, "[0;0;0;ran]"/1
  m_in|p/1 -> Demux4/1
  Demux4/1 -> Demux1/1
  W_./r_out|a/1 -> 6x6 v-u_rotation/1(u)
  Mux1/1 -> W_r_in/.|p/1
  Demux1/1 -> Mux/1
  Cm/1 -> Gain8/1, Sum4/2
  Demux/1 -> Mux1/1
  Gain2/1 -> Mux1/2
  Demux/2 -> Gain9/1
  Gain1/1 -> Mux2/2, Sum1/2
  Sum4/1 -> Gain1/1
  Gain3/1 -> Mux/2
  Demux3/2 -> Sum1/1
  Gain9/1 -> Demux2/1
  Demux2/2 -> Sum4/1
  Mux2/1 -> Gain3/1
  Demux1/2 -> Gain4/1
  Gain4/1 -> Demux3/1
  Mux3/1 -> Gain2/1
  Gain8/1 -> Mux3/2
  Demux2/1 -> Mux3/1
  Demux3/1 -> Mux2/1
  6x6 v-u_rotation/1(y) -> Demux/1
  18x18 v-u_rotation/1(y) -> m_out|a/1

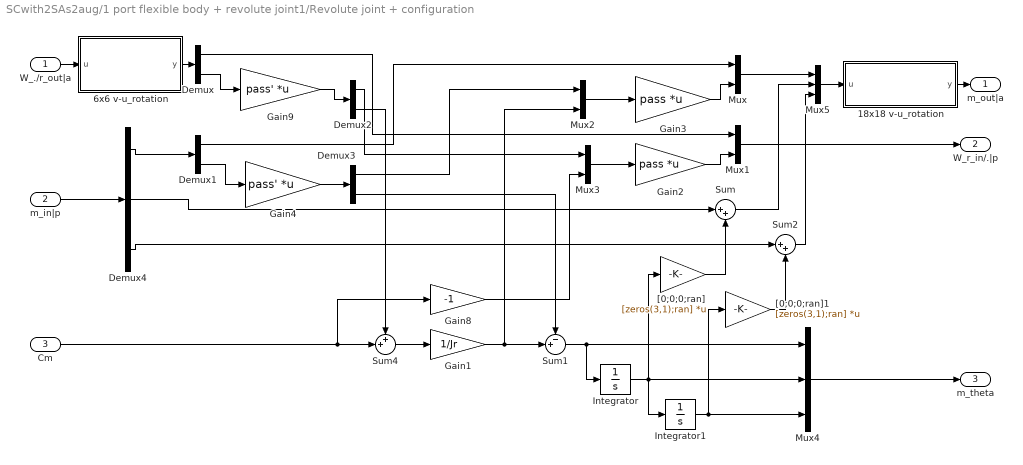
== system SCwith2SAs2aug/1 port flexible body + revolute joint1/Revolute joint + configuration ==
  W_./r_out|a : Inport  PortDimensions=6
  m_in|p : Inport  Port=2  PortDimensions=18
  Cm : Inport  Port=3  PortDimensions=1
  18x18 v-u_rotation : Subsystem  mask(18x18 rotation matrix (around a given axis)){ra=ra, theta=theta, transp=on}
      mask prompts: ra "Rotation axis (3x1 vector)"; theta "Angle (rad)"; transp "Matrix transposed"
      mask help:
      | For 6 d.o.f. body motion vector (3 translations and 3 rotations, acceleration velocities and positions), this block Implement the 18x18 rotation matrix (or its transposed)  for a given angle around a given axis.
      |
      | Angle  (rad) can be an uncertain parameter declared with "ureal" with mode 'Range'
      | Ex: ureal('NAME',0,'Range',[-pi pi])
      | Then, ULINEARIZE will provide a model involving the block named "tan_NAME_div4".
      mask init:
      | vUrotation3x3
      mask Help: web('Doc6vurotation.html','-browser')
      mask Display:
      | disp('v-rot\n18x18')
      | if transp
      |     port_label('input', 1, '[.]_R1')
      |     port_label('output', 1, '[.]_R2')
      | else
      |     port_label('input', 1, '[.]_R2')
      |     port_label('output', 1, '[.]_R1')
      | end
  6x6 v-u_rotation : Subsystem  mask(6x6 rotation matrix (around a given axis)){ra=ra, theta=theta, transp=off}
      mask prompts: ra "Rotation axis (3x1 vector)"; theta "Angle (rad)"; transp "Matrix transposed"
      mask help:
      | For 6 d.o.f. body motion (3 translations and 3 rotations), this block Implement the 6x6 rotation matrix (or its transposed) for a given angle around a given axis.
      |
      | Angle  (rad) can be an uncertain parameter declared with "ureal" with mode 'Range'
      | Ex: ureal('NAME',0,'Range',[-pi pi])
      | Then, ULINEARIZE will provide a model involving the block named "tan_NAME_div4".
      mask init:
      | vUrotation3x3
      mask Help: web('Doc6vurotation.html','-browser')
      mask Display:
      | disp('v-rot\n6x6')
      | if transp
      |     port_label('input', 1, '[.]_R1')
      |     port_label('output', 1, '[.]_R2')
      | else
      |     port_label('input', 1, '[.]_R2')
      |     port_label('output', 1, '[.]_R1')
      | end
  Demux : Demux  Outputs=[3 3]
  Demux1 : Demux  Outputs=[3 3]
  Demux2 : Demux  Outputs=[2 1]
  Demux3 : Demux  Outputs=[2 1]
  Demux4 : Demux  Outputs=[6 6 6]
  Gain1 : Gain  Gain=1/Jr
  Gain2 : Gain  Gain=pass  Multiplication=Matrix(K*u) (u vector)
  Gain3 : Gain  Gain=pass  Multiplication=Matrix(K*u) (u vector)
  Gain4 : Gain  Gain=pass'  Multiplication=Matrix(K*u) (u vector)
  Gain8 : Gain  Gain=-1
  Gain9 : Gain  Gain=pass'  Multiplication=Matrix(K*u) (u vector)
  Integrator : Integrator
  Integrator1 : Integrator
  Mux : Mux  Inputs=[3 3]
  Mux1 : Mux  Inputs=[3 3]
  Mux2 : Mux  Inputs=[2 1]
  Mux3 : Mux  Inputs=[2 1]
  Mux4 : Mux  Inputs=3
  Mux5 : Mux  Inputs=[6 6 6]
  Sum : Sum  Inputs=|++
  Sum1 : Sum  Inputs=-+|
  Sum2 : Sum  Inputs=|++
  Sum4 : Sum  Inputs=++|
  "[0;0;0;ran]" : Gain  Gain=[zeros(3,1);ran]  Multiplication=Matrix(K*u) (u vector)
  "[0;0;0;ran]1" : Gain  Gain=[zeros(3,1);ran]  Multiplication=Matrix(K*u) (u vector)
  m_out|a : Outport  VectorParamsAs1DForOutWhenUnconnected=off
  W_r_in/.|p : Outport  Port=2  VectorParamsAs1DForOutWhenUnconnected=off
  m_theta : Outport  Port=3  VectorParamsAs1DForOutWhenUnconnected=off
  wires:
  18x18 v-u_rotation/1(y) -> m_out|a/1
  6x6 v-u_rotation/1(y) -> Demux/1
  Demux3/1 -> Mux2/1
  Demux2/1 -> Mux3/1
  Gain8/1 -> Mux3/2
  Mux3/1 -> Gain2/1
  Gain4/1 -> Demux3/1
  Demux1/2 -> Gain4/1
  Mux2/1 -> Gain3/1
  Demux2/2 -> Sum4/1
  Gain9/1 -> Demux2/1
  Demux3/2 -> Sum1/1
  Gain3/1 -> Mux/2
  Sum4/1 -> Gain1/1
  Gain1/1 -> Sum1/2, Mux2/2
  Demux/2 -> Gain9/1
  Gain2/1 -> Mux1/2
  Demux/1 -> Mux1/1
  Cm/1 -> Sum4/2, Gain8/1
  Demux1/1 -> Mux/1
  Mux1/1 -> W_r_in/.|p/1
  W_./r_out|a/1 -> 6x6 v-u_rotation/1(u)
  Demux4/1 -> Demux1/1
  m_in|p/1 -> Demux4/1
  Integrator/1 -> "[0;0;0;ran]"/1, Mux4/2, Integrator1/1
  Mux4/1 -> m_theta/1
  Sum1/1 -> Integrator/1, Mux4/1
  Integrator1/1 -> "[0;0;0;ran]1"/1, Mux4/3
  "[0;0;0;ran]"/1 -> Sum/2
  "[0;0;0;ran]1"/1 -> Sum2/2
  Demux4/2 -> Sum/1
  Demux4/3 -> Sum2/1
  Mux/1 -> Mux5/1
  Mux5/1 -> 18x18 v-u_rotation/1(u)
  Sum/1 -> Mux5/2
  Sum2/1 -> Mux5/3

== system SCwith2SAs2aug/1 port flexible body + revolute joint/Revolute joint + configuration/18x18 v-u_rotation ==
  u : Inport  PortDimensions=18
  Demux : Demux  Outputs=[3 3 3 3 3 3]
  Mux : Mux  Inputs=[3 3 3 3 3 3]
  Subsystem : Subsystem
  Subsystem1 : Subsystem
  Subsystem2 : Subsystem
  Subsystem3 : Subsystem
  Subsystem4 : Subsystem
  Subsystem5 : Subsystem
  y : Outport  VectorParamsAs1DForOutWhenUnconnected=off
  wires:
  Subsystem5/1(Out1) -> Mux/6
  Demux/6 -> Subsystem5/1(In1)
  Subsystem4/1(Out1) -> Mux/5
  Demux/5 -> Subsystem4/1(In1)
  Subsystem3/1(Out1) -> Mux/4
  Demux/4 -> Subsystem3/1(In1)
  Subsystem2/1(Out1) -> Mux/3
  Demux/3 -> Subsystem2/1(In1)
  Mux/1 -> y/1
  u/1 -> Demux/1
  Demux/1 -> Subsystem/1(In1)
  Demux/2 -> Subsystem1/1(In1)
  Subsystem/1(Out1) -> Mux/1
  Subsystem1/1(Out1) -> Mux/2

== system SCwith2SAs2aug/1 port flexible body + revolute joint/Revolute joint + configuration/6x6 v-u_rotation ==
  u : Inport  PortDimensions=6
  Demux : Demux  Outputs=[3 3]
  Mux : Mux  Inputs=[3 3]
  Subsystem : Subsystem
  Subsystem1 : Subsystem
  y : Outport  VectorParamsAs1DForOutWhenUnconnected=off
  wires:
  Subsystem1/1(Out1) -> Mux/2
  Subsystem/1(Out1) -> Mux/1
  Demux/2 -> Subsystem1/1(In1)
  Demux/1 -> Subsystem/1(In1)
  u/1 -> Demux/1
  Mux/1 -> y/1

== system SCwith2SAs2aug/1 port flexible body + revolute joint1/Revolute joint + configuration/18x18 v-u_rotation ==
  u : Inport  PortDimensions=18
  Demux : Demux  Outputs=[3 3 3 3 3 3]
  Mux : Mux  Inputs=[3 3 3 3 3 3]
  Subsystem : Subsystem
  Subsystem1 : Subsystem
  Subsystem2 : Subsystem
  Subsystem3 : Subsystem
  Subsystem4 : Subsystem
  Subsystem5 : Subsystem
  y : Outport  VectorParamsAs1DForOutWhenUnconnected=off
  wires:
  Subsystem1/1(Out1) -> Mux/2
  Subsystem/1(Out1) -> Mux/1
  Demux/2 -> Subsystem1/1(In1)
  Demux/1 -> Subsystem/1(In1)
  u/1 -> Demux/1
  Mux/1 -> y/1
  Demux/3 -> Subsystem2/1(In1)
  Subsystem2/1(Out1) -> Mux/3
  Demux/4 -> Subsystem3/1(In1)
  Subsystem3/1(Out1) -> Mux/4
  Demux/5 -> Subsystem4/1(In1)
  Subsystem4/1(Out1) -> Mux/5
  Demux/6 -> Subsystem5/1(In1)
  Subsystem5/1(Out1) -> Mux/6

== system SCwith2SAs2aug/1 port flexible body + revolute joint1/Revolute joint + configuration/6x6 v-u_rotation ==
  u : Inport  PortDimensions=6
  Demux : Demux  Outputs=[3 3]
  Mux : Mux  Inputs=[3 3]
  Subsystem : Subsystem
  Subsystem1 : Subsystem
  y : Outport  VectorParamsAs1DForOutWhenUnconnected=off
  wires:
  Mux/1 -> y/1
  u/1 -> Demux/1
  Demux/1 -> Subsystem/1(In1)
  Demux/2 -> Subsystem1/1(In1)
  Subsystem/1(Out1) -> Mux/1
  Subsystem1/1(Out1) -> Mux/2

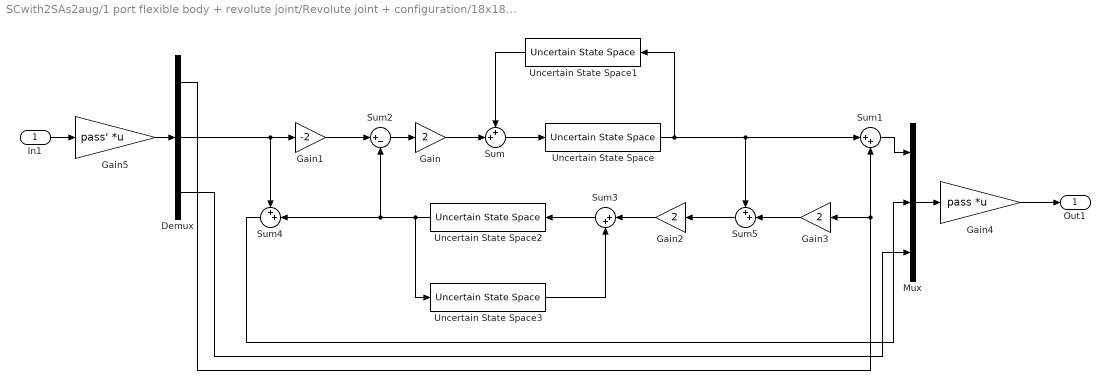
== system SCwith2SAs2aug/1 port flexible body + revolute joint/Revolute joint + configuration/18x18 v-u_rotation/Subsystem ==
  In1 : Inport
  Demux : Demux  Outputs=3
  Gain : Gain  Gain=2
  Gain1 : Gain  Gain=-2
  Gain2 : Gain  Gain=2
  Gain3 : Gain  Gain=2
  Gain4 : Gain  Gain=pass  Multiplication=Matrix(K*u) (u vector)
  Gain5 : Gain  Gain=pass'  Multiplication=Matrix(K*u) (u vector)
  Mux : Mux  Inputs=3
  Sum : Sum  Inputs=++|
  Sum1 : Sum  Inputs=|++
  Sum2 : Sum  Inputs=|+-
  Sum3 : Sum  Inputs=|++
  Sum4 : Sum  Inputs=++|
  Sum5 : Sum  Inputs=++|
  Uncertain State Space{,1..3} (4 alike) : RCTblocks/Uncertain State Space  Tag=USS  USystem=uss(sig4)  UValue=[]  X0=[]  uX0=[]
  Out1 : Outport  VectorParamsAs1DForOutWhenUnconnected=off
  wires:
  Sum5/1 -> Gain2/1
  Sum1/1 -> Mux/1
  Sum2/1 -> Gain/1
  Uncertain State Space1/1 -> Sum/1
  Demux/2 -> Gain1/1, Sum4/1
  Sum/1 -> Uncertain State Space/1
  Gain3/1 -> Sum5/2
  Uncertain State Space/1 -> Sum1/1, Sum5/1, Uncertain State Space1/1
  Gain1/1 -> Sum2/1
  Sum3/1 -> Uncertain State Space2/1
  Sum4/1 -> Mux/2
  Mux/1 -> Gain4/1
  Demux/3 -> Mux/3
  Demux/1 -> Sum1/2, Gain3/1
  Uncertain State Space2/1 -> Sum2/2, Sum4/2, Uncertain State Space3/1
  Gain/1 -> Sum/2
  In1/1 -> Gain5/1
  Gain2/1 -> Sum3/1
  Uncertain State Space3/1 -> Sum3/2
  Gain4/1 -> Out1/1
  Gain5/1 -> Demux/1

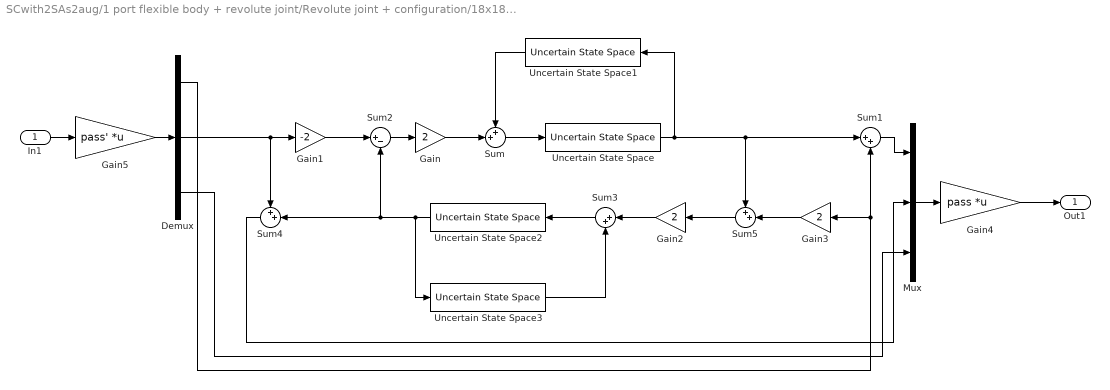
== system SCwith2SAs2aug/1 port flexible body + revolute joint/Revolute joint + configuration/18x18 v-u_rotation/Subsystem1 ==
  In1 : Inport
  Demux : Demux  Outputs=3
  Gain : Gain  Gain=2
  Gain1 : Gain  Gain=-2
  Gain2 : Gain  Gain=2
  Gain3 : Gain  Gain=2
  Gain4 : Gain  Gain=pass  Multiplication=Matrix(K*u) (u vector)
  Gain5 : Gain  Gain=pass'  Multiplication=Matrix(K*u) (u vector)
  Mux : Mux  Inputs=3
  Sum : Sum  Inputs=++|
  Sum1 : Sum  Inputs=|++
  Sum2 : Sum  Inputs=|+-
  Sum3 : Sum  Inputs=|++
  Sum4 : Sum  Inputs=++|
  Sum5 : Sum  Inputs=++|
  Uncertain State Space{,1..3} (4 alike) : RCTblocks/Uncertain State Space  Tag=USS  USystem=uss(sig4)  UValue=[]  X0=[]  uX0=[]
  Out1 : Outport  VectorParamsAs1DForOutWhenUnconnected=off
  wires:
  Gain4/1 -> Out1/1
  Uncertain State Space3/1 -> Sum3/2
  Gain2/1 -> Sum3/1
  In1/1 -> Gain5/1
  Gain/1 -> Sum/2
  Uncertain State Space2/1 -> Uncertain State Space3/1, Sum4/2, Sum2/2
  Demux/1 -> Gain3/1, Sum1/2
  Demux/3 -> Mux/3
  Mux/1 -> Gain4/1
  Sum4/1 -> Mux/2
  Sum3/1 -> Uncertain State Space2/1
  Gain1/1 -> Sum2/1
  Uncertain State Space/1 -> Uncertain State Space1/1, Sum5/1, Sum1/1
  Gain3/1 -> Sum5/2
  Sum/1 -> Uncertain State Space/1
  Demux/2 -> Sum4/1, Gain1/1
  Uncertain State Space1/1 -> Sum/1
  Sum2/1 -> Gain/1
  Sum1/1 -> Mux/1
  Sum5/1 -> Gain2/1
  Gain5/1 -> Demux/1

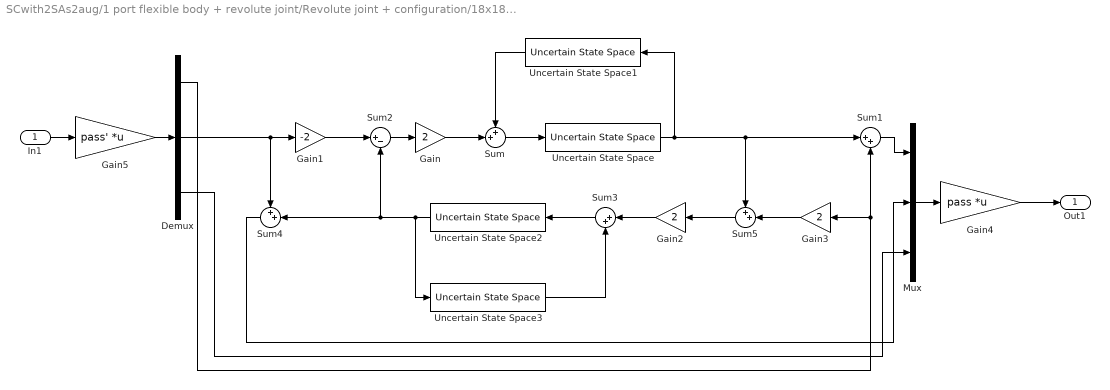
== system SCwith2SAs2aug/1 port flexible body + revolute joint/Revolute joint + configuration/18x18 v-u_rotation/Subsystem2 ==
  In1 : Inport
  Demux : Demux  Outputs=3
  Gain : Gain  Gain=2
  Gain1 : Gain  Gain=-2
  Gain2 : Gain  Gain=2
  Gain3 : Gain  Gain=2
  Gain4 : Gain  Gain=pass  Multiplication=Matrix(K*u) (u vector)
  Gain5 : Gain  Gain=pass'  Multiplication=Matrix(K*u) (u vector)
  Mux : Mux  Inputs=3
  Sum : Sum  Inputs=++|
  Sum1 : Sum  Inputs=|++
  Sum2 : Sum  Inputs=|+-
  Sum3 : Sum  Inputs=|++
  Sum4 : Sum  Inputs=++|
  Sum5 : Sum  Inputs=++|
  Uncertain State Space{,1..3} (4 alike) : RCTblocks/Uncertain State Space  Tag=USS  USystem=uss(sig4)  UValue=[]  X0=[]  uX0=[]
  Out1 : Outport  VectorParamsAs1DForOutWhenUnconnected=off
  wires:
  Gain5/1 -> Demux/1
  Gain4/1 -> Out1/1
  Uncertain State Space3/1 -> Sum3/2
  Gain2/1 -> Sum3/1
  In1/1 -> Gain5/1
  Gain/1 -> Sum/2
  Uncertain State Space2/1 -> Uncertain State Space3/1, Sum4/2, Sum2/2
  Demux/1 -> Gain3/1, Sum1/2
  Demux/3 -> Mux/3
  Mux/1 -> Gain4/1
  Sum4/1 -> Mux/2
  Sum3/1 -> Uncertain State Space2/1
  Gain1/1 -> Sum2/1
  Uncertain State Space/1 -> Uncertain State Space1/1, Sum5/1, Sum1/1
  Gain3/1 -> Sum5/2
  Sum/1 -> Uncertain State Space/1
  Demux/2 -> Sum4/1, Gain1/1
  Uncertain State Space1/1 -> Sum/1
  Sum2/1 -> Gain/1
  Sum1/1 -> Mux/1
  Sum5/1 -> Gain2/1

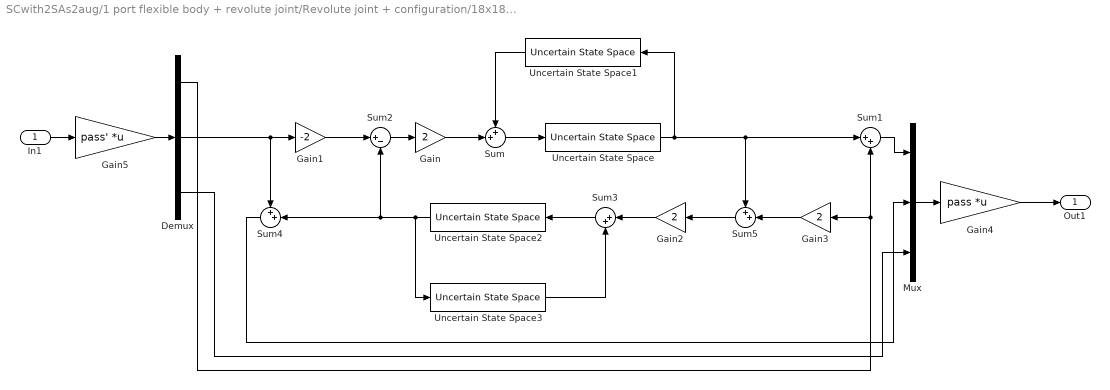
== system SCwith2SAs2aug/1 port flexible body + revolute joint/Revolute joint + configuration/18x18 v-u_rotation/Subsystem3 ==
  In1 : Inport
  Demux : Demux  Outputs=3
  Gain : Gain  Gain=2
  Gain1 : Gain  Gain=-2
  Gain2 : Gain  Gain=2
  Gain3 : Gain  Gain=2
  Gain4 : Gain  Gain=pass  Multiplication=Matrix(K*u) (u vector)
  Gain5 : Gain  Gain=pass'  Multiplication=Matrix(K*u) (u vector)
  Mux : Mux  Inputs=3
  Sum : Sum  Inputs=++|
  Sum1 : Sum  Inputs=|++
  Sum2 : Sum  Inputs=|+-
  Sum3 : Sum  Inputs=|++
  Sum4 : Sum  Inputs=++|
  Sum5 : Sum  Inputs=++|
  Uncertain State Space{,1..3} (4 alike) : RCTblocks/Uncertain State Space  Tag=USS  USystem=uss(sig4)  UValue=[]  X0=[]  uX0=[]
  Out1 : Outport  VectorParamsAs1DForOutWhenUnconnected=off
  wires:
  Gain5/1 -> Demux/1
  Sum5/1 -> Gain2/1
  Sum1/1 -> Mux/1
  Sum2/1 -> Gain/1
  Uncertain State Space1/1 -> Sum/1
  Demux/2 -> Gain1/1, Sum4/1
  Sum/1 -> Uncertain State Space/1
  Gain3/1 -> Sum5/2
  Uncertain State Space/1 -> Sum1/1, Sum5/1, Uncertain State Space1/1
  Gain1/1 -> Sum2/1
  Sum3/1 -> Uncertain State Space2/1
  Sum4/1 -> Mux/2
  Mux/1 -> Gain4/1
  Demux/3 -> Mux/3
  Demux/1 -> Sum1/2, Gain3/1
  Uncertain State Space2/1 -> Sum2/2, Sum4/2, Uncertain State Space3/1
  Gain/1 -> Sum/2
  In1/1 -> Gain5/1
  Gain2/1 -> Sum3/1
  Uncertain State Space3/1 -> Sum3/2
  Gain4/1 -> Out1/1

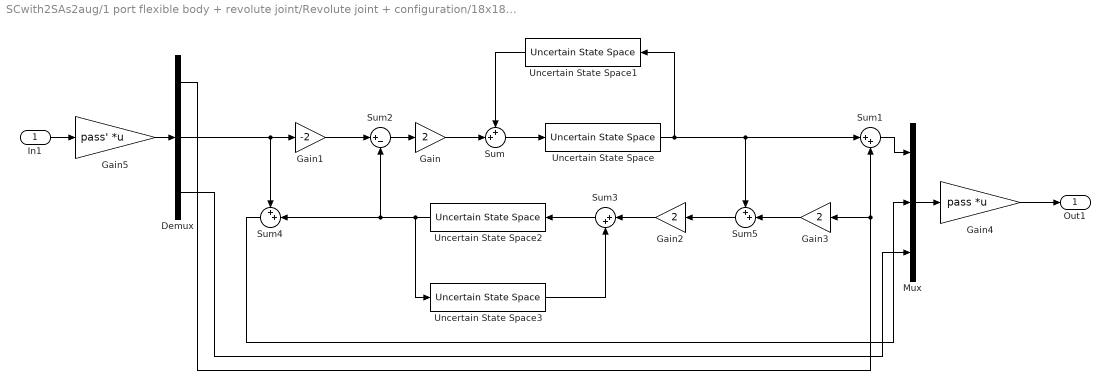
== system SCwith2SAs2aug/1 port flexible body + revolute joint/Revolute joint + configuration/18x18 v-u_rotation/Subsystem4 ==
  In1 : Inport
  Demux : Demux  Outputs=3
  Gain : Gain  Gain=2
  Gain1 : Gain  Gain=-2
  Gain2 : Gain  Gain=2
  Gain3 : Gain  Gain=2
  Gain4 : Gain  Gain=pass  Multiplication=Matrix(K*u) (u vector)
  Gain5 : Gain  Gain=pass'  Multiplication=Matrix(K*u) (u vector)
  Mux : Mux  Inputs=3
  Sum : Sum  Inputs=++|
  Sum1 : Sum  Inputs=|++
  Sum2 : Sum  Inputs=|+-
  Sum3 : Sum  Inputs=|++
  Sum4 : Sum  Inputs=++|
  Sum5 : Sum  Inputs=++|
  Uncertain State Space{,1..3} (4 alike) : RCTblocks/Uncertain State Space  Tag=USS  USystem=uss(sig4)  UValue=[]  X0=[]  uX0=[]
  Out1 : Outport  VectorParamsAs1DForOutWhenUnconnected=off
  wires:
  Sum5/1 -> Gain2/1
  Sum1/1 -> Mux/1
  Sum2/1 -> Gain/1
  Uncertain State Space1/1 -> Sum/1
  Demux/2 -> Gain1/1, Sum4/1
  Sum/1 -> Uncertain State Space/1
  Gain3/1 -> Sum5/2
  Uncertain State Space/1 -> Sum1/1, Sum5/1, Uncertain State Space1/1
  Gain1/1 -> Sum2/1
  Sum3/1 -> Uncertain State Space2/1
  Sum4/1 -> Mux/2
  Mux/1 -> Gain4/1
  Demux/3 -> Mux/3
  Demux/1 -> Sum1/2, Gain3/1
  Uncertain State Space2/1 -> Sum2/2, Sum4/2, Uncertain State Space3/1
  Gain/1 -> Sum/2
  In1/1 -> Gain5/1
  Gain2/1 -> Sum3/1
  Uncertain State Space3/1 -> Sum3/2
  Gain4/1 -> Out1/1
  Gain5/1 -> Demux/1

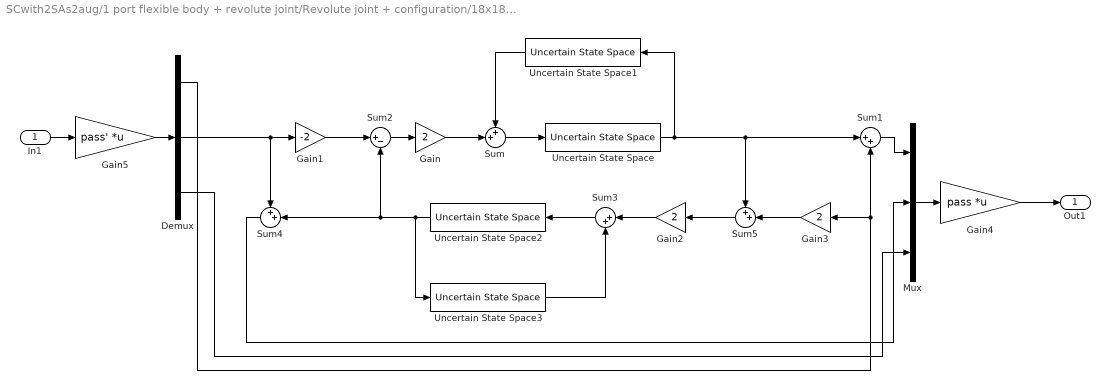
== system SCwith2SAs2aug/1 port flexible body + revolute joint/Revolute joint + configuration/18x18 v-u_rotation/Subsystem5 ==
  In1 : Inport
  Demux : Demux  Outputs=3
  Gain : Gain  Gain=2
  Gain1 : Gain  Gain=-2
  Gain2 : Gain  Gain=2
  Gain3 : Gain  Gain=2
  Gain4 : Gain  Gain=pass  Multiplication=Matrix(K*u) (u vector)
  Gain5 : Gain  Gain=pass'  Multiplication=Matrix(K*u) (u vector)
  Mux : Mux  Inputs=3
  Sum : Sum  Inputs=++|
  Sum1 : Sum  Inputs=|++
  Sum2 : Sum  Inputs=|+-
  Sum3 : Sum  Inputs=|++
  Sum4 : Sum  Inputs=++|
  Sum5 : Sum  Inputs=++|
  Uncertain State Space{,1..3} (4 alike) : RCTblocks/Uncertain State Space  Tag=USS  USystem=uss(sig4)  UValue=[]  X0=[]  uX0=[]
  Out1 : Outport  VectorParamsAs1DForOutWhenUnconnected=off
  wires:
  Gain4/1 -> Out1/1
  Uncertain State Space3/1 -> Sum3/2
  Gain2/1 -> Sum3/1
  In1/1 -> Gain5/1
  Gain/1 -> Sum/2
  Uncertain State Space2/1 -> Uncertain State Space3/1, Sum4/2, Sum2/2
  Demux/1 -> Gain3/1, Sum1/2
  Demux/3 -> Mux/3
  Mux/1 -> Gain4/1
  Sum4/1 -> Mux/2
  Sum3/1 -> Uncertain State Space2/1
  Gain1/1 -> Sum2/1
  Uncertain State Space/1 -> Uncertain State Space1/1, Sum5/1, Sum1/1
  Gain3/1 -> Sum5/2
  Sum/1 -> Uncertain State Space/1
  Demux/2 -> Sum4/1, Gain1/1
  Uncertain State Space1/1 -> Sum/1
  Sum2/1 -> Gain/1
  Sum1/1 -> Mux/1
  Sum5/1 -> Gain2/1
  Gain5/1 -> Demux/1

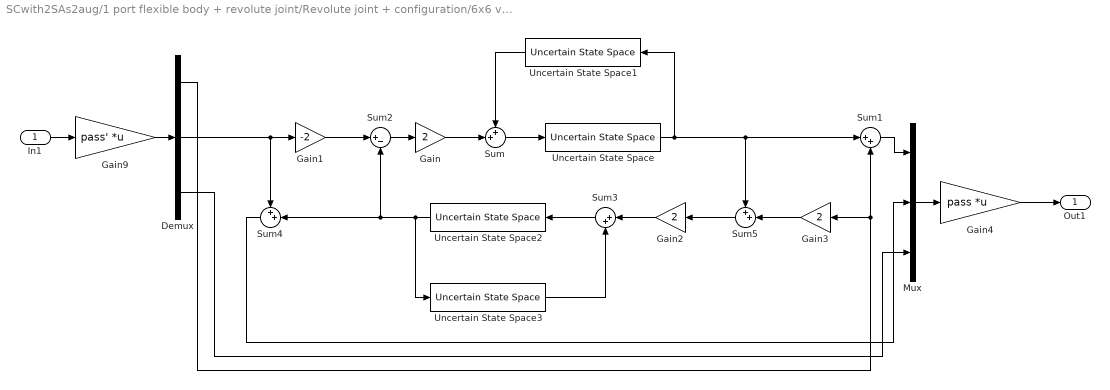
== system SCwith2SAs2aug/1 port flexible body + revolute joint/Revolute joint + configuration/6x6 v-u_rotation/Subsystem ==
  In1 : Inport
  Demux : Demux  Outputs=3
  Gain : Gain  Gain=2
  Gain1 : Gain  Gain=-2
  Gain2 : Gain  Gain=2
  Gain3 : Gain  Gain=2
  Gain4 : Gain  Gain=pass  Multiplication=Matrix(K*u) (u vector)
  Gain9 : Gain  Gain=pass'  Multiplication=Matrix(K*u) (u vector)
  Mux : Mux  Inputs=3
  Sum : Sum  Inputs=++|
  Sum1 : Sum  Inputs=|++
  Sum2 : Sum  Inputs=|+-
  Sum3 : Sum  Inputs=|++
  Sum4 : Sum  Inputs=++|
  Sum5 : Sum  Inputs=++|
  Uncertain State Space{,1..3} (4 alike) : RCTblocks/Uncertain State Space  Tag=USS  USystem=uss(sig4)  UValue=[]  X0=[]  uX0=[]
  Out1 : Outport  VectorParamsAs1DForOutWhenUnconnected=off
  wires:
  Gain4/1 -> Out1/1
  Uncertain State Space3/1 -> Sum3/2
  Gain2/1 -> Sum3/1
  Gain9/1 -> Demux/1
  Gain/1 -> Sum/2
  Uncertain State Space2/1 -> Uncertain State Space3/1, Sum4/2, Sum2/2
  Demux/1 -> Gain3/1, Sum1/2
  Demux/3 -> Mux/3
  Mux/1 -> Gain4/1
  In1/1 -> Gain9/1
  Sum4/1 -> Mux/2
  Sum3/1 -> Uncertain State Space2/1
  Gain1/1 -> Sum2/1
  Uncertain State Space/1 -> Uncertain State Space1/1, Sum5/1, Sum1/1
  Gain3/1 -> Sum5/2
  Sum/1 -> Uncertain State Space/1
  Demux/2 -> Sum4/1, Gain1/1
  Uncertain State Space1/1 -> Sum/1
  Sum2/1 -> Gain/1
  Sum1/1 -> Mux/1
  Sum5/1 -> Gain2/1
